simulink model "cascaded_pid_impedance_torque"  (R2015a)
settings: Solver=ode45  StartTime=0.0  StopTime=10.0  RelTol=1e-3
libraries: simulink x1
settings Model: Creator=preston  LastModifiedBy=preston

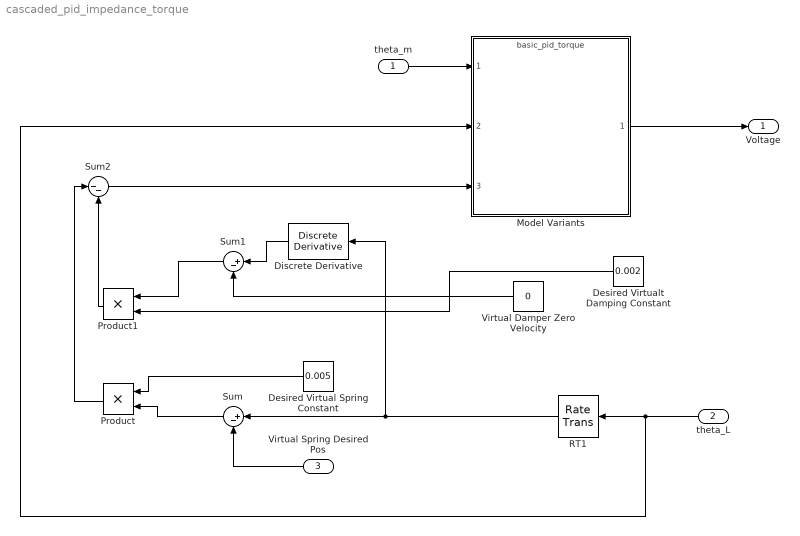
== system cascaded_pid_impedance_torque ==
  theta_m : Inport
  theta_L : Inport  Port=2
  Virtual Spring Desired Pos : Inport  Port=3
  "Desired Virtual Spring Constant " : Constant  Value=0.005
  "Desired Virtualt Damping Constant " : Constant  Value=0.002
  Discrete Derivative : simulink/Discrete/Discrete Derivative  gainval=1.0  ICPrevScaledInput=0.0  InputProcessing=Inherited  OutMin=[]  OutMax=[]  OutDataType=fixdt(1, 16)  OutScaling=2^-10  DoSatur=off
  Model Variants : ModelReference  ModelNameDialog=basic_pid_torque.slx  SimulationMode=Normal  ModelReferenceVersion=1.23  CopyOfModelName=basic_pid_torque.slx  DefaultDataLogging=on
      settings: AttributesFormatString=%<ActiveVariant>
  Product : Product
  Product1 : Product
  RT1 : RateTransition  OutPortSampleTime=T_sample_control
  Sum : Sum  Inputs=|+-
  Sum1 : Sum  Inputs=|+-
  Sum2 : Sum  Inputs=|--
  Virtual Damper Zero Velocity : Constant  Value=0
  Voltage : Outport
  wires:
  theta_L/1 -> Model Variants/2, RT1/1
  RT1/1 -> Sum/1, Discrete Derivative/1
  Sum/1 -> Product/2
  "Desired Virtual Spring Constant "/1 -> Product/1
  Discrete Derivative/1 -> Sum1/1
  Virtual Damper Zero Velocity/1 -> Sum1/2
  "Desired Virtualt Damping Constant "/1 -> Product1/2
  Sum1/1 -> Product1/1
  Product1/1 -> Sum2/2
  Product/1 -> Sum2/1
  Sum2/1 -> Model Variants/3
  Model Variants/1 -> Voltage/1
  theta_m/1 -> Model Variants/1
  Virtual Spring Desired Pos/1 -> Sum/2
